simulink model "Lorenz"  (R2016a)
settings: Solver=VariableStepAuto  StartTime=0.0  StopTime=100  RelTol=1e-3
values from neighbouring files (symbols this model uses):
  b = 8/3    (= 2.66666666667)    [fct5.m]
  r = 28    [fct5.m]
  rho = 10    [fct5.m]
settings Model: Creator=Cds  LastModifiedBy=Cds
settings GRTTargetCC: GeneratePreprocessorConditionals=Use local settings

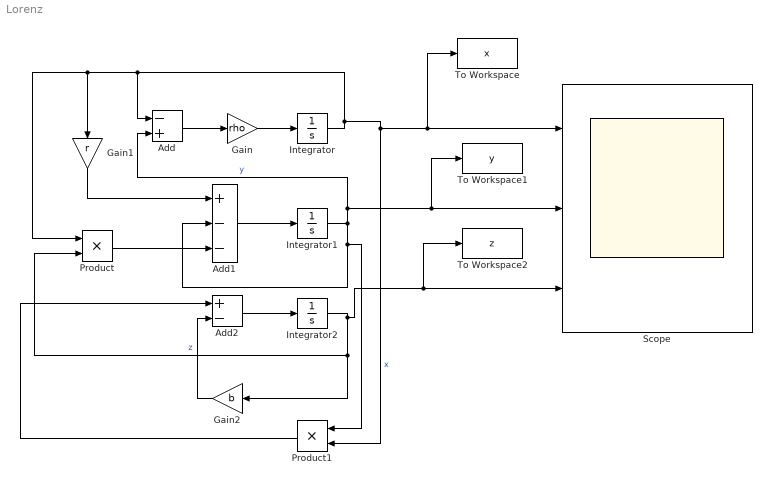
== system Lorenz ==
  Add : Sum  Inputs=-+
  Add1 : Sum  Inputs=+--
  Add2 : Sum  Inputs=+-
  Gain : Gain  Gain=rho
  Gain1 : Gain  Gain=r
  Gain2 : Gain  Gain=b
  Integrator : Integrator  InitialCondition=.1
  Integrator1 : Integrator  InitialCondition=.1
  Integrator2 : Integrator  InitialCondition=.1
  Product : Product
  Product1 : Product
  Scope : Scope  NumInputPorts=3
  To Workspace : ToWorkspace  VariableName=x  SampleTime=-1
      settings: Save2DSignal=2-D array (concatenate along first dimension)
  To Workspace1 : ToWorkspace  VariableName=y  SampleTime=-1
      settings: Save2DSignal=2-D array (concatenate along first dimension)
  To Workspace2 : ToWorkspace  VariableName=z  SampleTime=-1
      settings: Save2DSignal=2-D array (concatenate along first dimension)
  wires:
  Gain/1 -> Integrator/1
  Add/1 -> Gain/1
  Integrator/1 -> To Workspace/1, Scope/1, Product1/2, Add/1, Gain1/1, Product/1  "x"
  Integrator1/1 -> To Workspace1/1, Scope/2, Add/2, Product1/1, Add1/2  "y"
  Add1/1 -> Integrator1/1
  Gain1/1 -> Add1/1
  Integrator2/1 -> To Workspace2/1, Scope/3, Gain2/1, Product/2  "z"
  Product/1 -> Add1/3
  Add2/1 -> Integrator2/1
  Product1/1 -> Add2/1
  Gain2/1 -> Add2/2
